simulink model "RoomModel"  (R2018a)
settings: Solver=VariableStepAuto  StartTime=0.0  StopTime=24  RelTol=1e-3
settings Model: Creator=jim  LastModifiedBy=jim

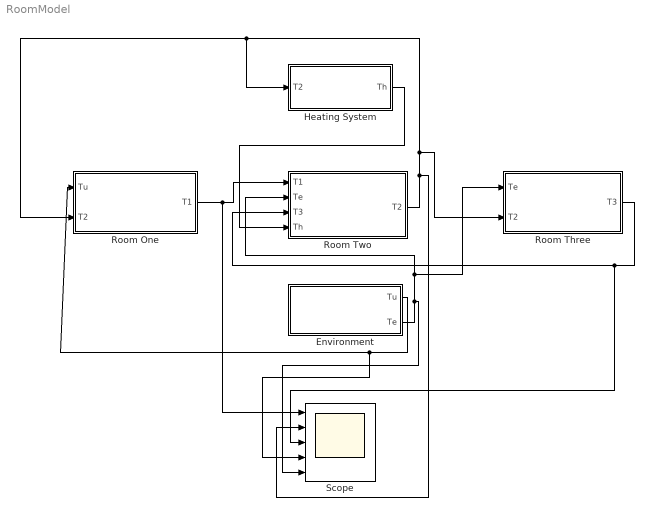
== system RoomModel ==
  Environment : Subsystem
  Heating System : Subsystem
  Room One : Subsystem
  Room Three : Subsystem
  Room Two : Subsystem
  Scope : Scope  NumInputPorts=5
  wires:
  Environment/1(Tu) -> Scope/4, Room One/1(Tu)
  Room One/1(T1) -> Scope/1, Room Two/1(T1)
  Environment/2("Te ") -> Scope/5, Room Three/1(Te), Room Two/2(Te)
  Heating System/1(Th) -> Room Two/4(Th)
  Room Two/1(T2) -> Scope/2, Room Three/2(T2), Room One/2(T2), Heating System/1(T2)
  Room Three/1(T3) -> Scope/3, Room Two/3(T3)

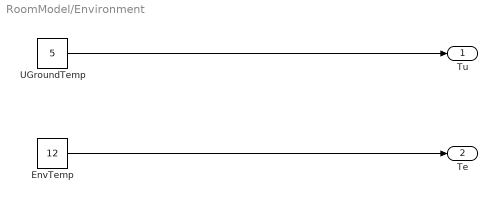
== system RoomModel/Environment ==
  EnvTemp : Constant  Value=12
  UGroundTemp : Constant  Value=5
  Tu : Outport
  "Te " : Outport  Port=2
  wires:
  UGroundTemp/1 -> Tu/1
  EnvTemp/1 -> "Te "/1

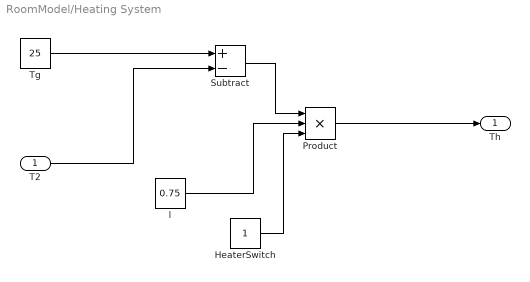
== system RoomModel/Heating System ==
  T2 : Inport
  HeaterSwitch : Constant
  Product : Product  Inputs=3
  Subtract : Sum  Inputs=+-
  Tg : Constant  Value=25
  l : Constant  Value=0.75
  Th : Outport
  wires:
  T2/1 -> Subtract/2
  Tg/1 -> Subtract/1
  Subtract/1 -> Product/1
  l/1 -> Product/2
  Product/1 -> Th/1
  HeaterSwitch/1 -> Product/3

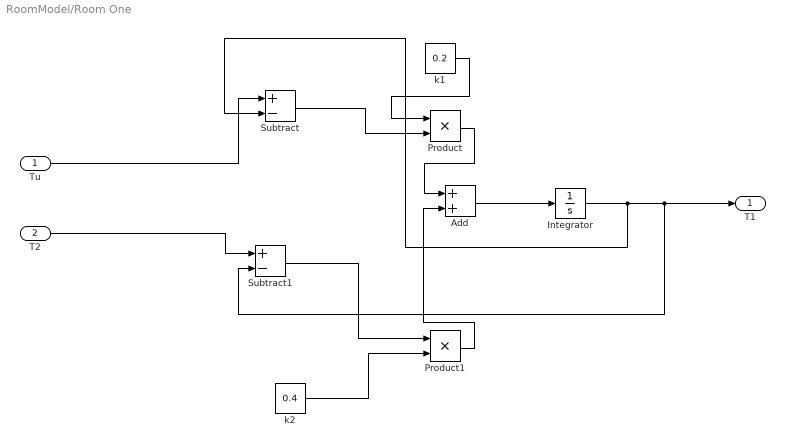
== system RoomModel/Room One ==
  Tu : Inport
  T2 : Inport  Port=2
  Add : Sum
  Integrator : Integrator  InitialCondition=10
  Product : Product
  Product1 : Product
  Subtract : Sum  Inputs=+-
  Subtract1 : Sum  Inputs=+-
  k1 : Constant  Value=0.2
  k2 : Constant  Value=0.4
  T1 : Outport
  wires:
  Tu/1 -> Subtract/1
  Integrator/1 -> Subtract/2, Subtract1/2, T1/1
  Subtract/1 -> Product/2
  k1/1 -> Product/1
  Add/1 -> Integrator/1
  Product/1 -> Add/1
  T2/1 -> Subtract1/1
  k2/1 -> Product1/2
  Subtract1/1 -> Product1/1
  Product1/1 -> Add/2

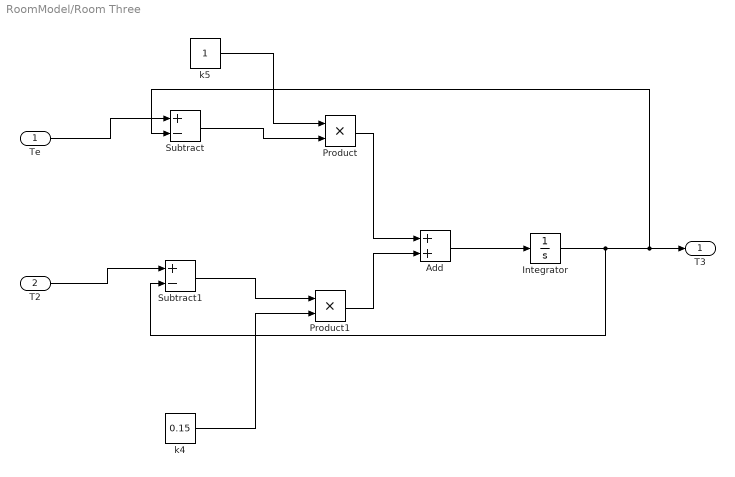
== system RoomModel/Room Three ==
  Te : Inport
  T2 : Inport  Port=2
  Add : Sum
  Integrator : Integrator  InitialCondition=15
  Product : Product
  Product1 : Product
  Subtract : Sum  Inputs=+-
  Subtract1 : Sum  Inputs=+-
  k4 : Constant  Value=0.15
  k5 : Constant
  T3 : Outport
  wires:
  Integrator/1 -> Subtract1/2, Subtract/2, T3/1
  Add/1 -> Integrator/1
  Product/1 -> Add/1
  Product1/1 -> Add/2
  k4/1 -> Product1/2
  Subtract1/1 -> Product1/1
  T2/1 -> Subtract1/1
  Te/1 -> Subtract/1
  k5/1 -> Product/1
  Subtract/1 -> Product/2

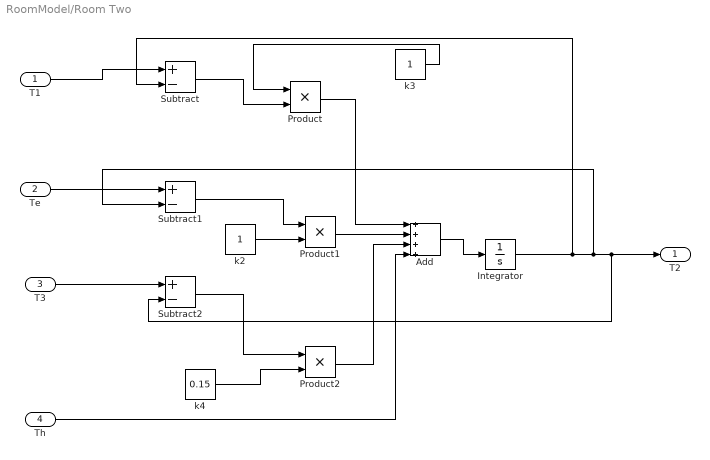
== system RoomModel/Room Two ==
  T1 : Inport
  Te : Inport  Port=2
  T3 : Inport  Port=3
  Th : Inport  Port=4
  Add : Sum  Inputs=++++
  Integrator : Integrator  InitialCondition=15
  Product : Product
  Product1 : Product
  Product2 : Product
  Subtract : Sum  Inputs=+-
  Subtract1 : Sum  Inputs=+-
  Subtract2 : Sum  Inputs=+-
  k2 : Constant
  k3 : Constant
  k4 : Constant  Value=0.15
  T2 : Outport
  wires:
  Integrator/1 -> Subtract/2, Subtract1/2, Subtract2/2, T2/1
  Add/1 -> Integrator/1
  Th/1 -> Add/4
  T1/1 -> Subtract/1
  Te/1 -> Subtract1/1
  T3/1 -> Subtract2/1
  Subtract/1 -> Product/2
  k3/1 -> Product/1
  Product/1 -> Add/1
  Product1/1 -> Add/2
  Product2/1 -> Add/3
  Subtract2/1 -> Product2/1
  k4/1 -> Product2/2
  k2/1 -> Product1/2
  Subtract1/1 -> Product1/1
